simulink model "Performance_Blocks"  (R2015b)
settings: Solver=VariableStepAuto  StartTime=0.0  StopTime=10.0  RelTol=1e-3
libraries: simulink x2
settings Model: Creator=Bogdan.Borowy  LastModifiedBy=Bogdan.Borowy

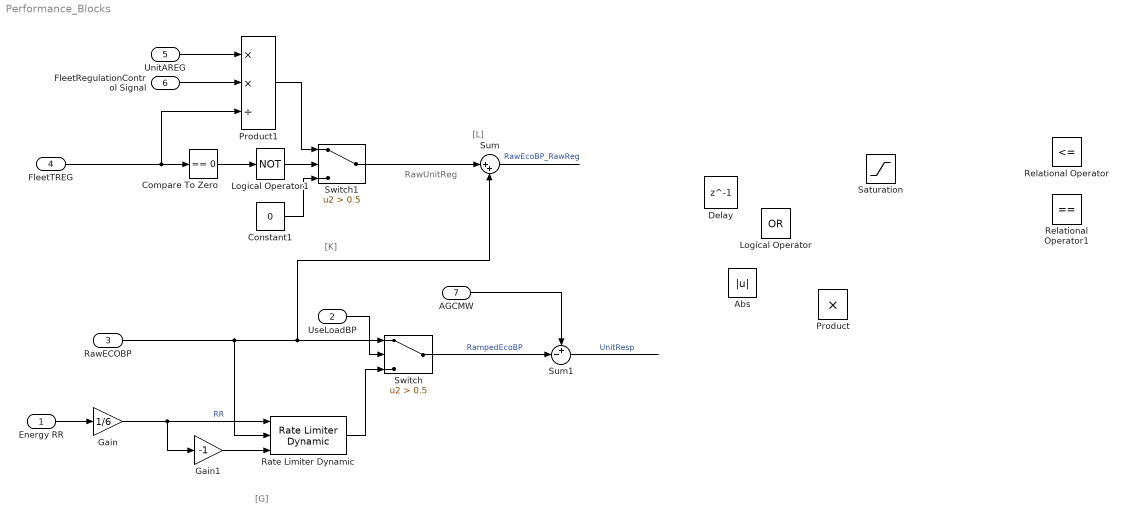
== system Performance_Blocks ==
  note: [L]
  note: [K]
  note: RawUnitReg
  note: [G]
  Energy RR : Inport
  UseLoadBP : Inport  Port=2
  RawECOBP : Inport  Port=3
  FleetTREG : Inport  Port=4
  UnitAREG : Inport  Port=5
  FleetRegulationControl Signal : Inport  Port=6
  AGCMW : Inport  Port=7
  Abs : Abs
  Compare To Zero : simulink/Logic and Bit Operations/Compare To Zero  relop===  OutDataTypeStr=boolean
  Constant1 : Constant  Value=0
  Delay : Delay  DelayLength=1  InitialCondition=0
  Gain : Gain  Gain=1/6
  Gain1 : Gain  Gain=-1
  Logical Operator : Logic  Operator=OR  AllPortsSameDT=off  OutDataTypeStr=boolean
  Logical Operator1 : Logic  Operator=NOT  AllPortsSameDT=off  OutDataTypeStr=boolean
  Product : Product
  Product1 : Product  Inputs=**/
  Rate Limiter Dynamic : simulink/Discontinuities/Rate Limiter Dynamic
  Relational Operator : RelationalOperator  Operator=<=  OutDataTypeStr=boolean
  Relational Operator1 : RelationalOperator  Operator===  OutDataTypeStr=boolean
  Saturation : Saturate
  Sum : Sum  Inputs=|++
  Sum1 : Sum  Inputs=+-|
  Switch : Switch  Criteria=u2 > Threshold  Threshold=0.5
  Switch1 : Switch  Criteria=u2 > Threshold  Threshold=0.5
  wires:
  Energy RR/1 -> Gain/1
  Gain/1 -> Gain1/1, Rate Limiter Dynamic/1  "RR"
  UseLoadBP/1 -> Switch/2
  Gain1/1 -> Rate Limiter Dynamic/3
  Rate Limiter Dynamic/1 -> Switch/3
  Compare To Zero/1 -> Logical Operator1/1
  FleetTREG/1 -> Product1/3, Compare To Zero/1
  Logical Operator1/1 -> Switch1/2
  Constant1/1 -> Switch1/3
  UnitAREG/1 -> Product1/1
  FleetRegulationControl Signal/1 -> Product1/2
  Product1/1 -> Switch1/1
  Switch1/1 -> Sum/1
  RawECOBP/1 -> Rate Limiter Dynamic/2, Sum/2, Switch/1
  Sum/1 -> ?  "RawEcoBP_RawReg"
  Switch/1 -> Sum1/2  "RampedEcoBP"
  AGCMW/1 -> Sum1/1
  Sum1/1 -> ?  "UnitResp"
